simulink model "SURVEY_Simulations"  (R2021b)
settings: Solver=ode4  StartTime=0.0  StopTime=60  FixedStep=1e-3  RelTol=1e-3
(part 2 of 2)

== matlab function SURVEY_Simulations/Desired Trajectory ==
  data: t input; p_d output; dot_p_d output; ddot_p_d output; psi_d output; delta_p output; delta_eta output
function [p_d, dot_p_d, ddot_p_d, psi_d, delta_p, delta_eta] = fcn(t)
z0    = 0.3;
h     = 1.4;
%% Circunferencia
% ampx = 1;
% ampy = 1;
% ampz = 0.1;
% amps = 10*pi/180;
% frecx = 2*pi/5;
% frecy = 2*pi/5;
% frecz = 2*pi/5;
% frecs = 2*pi/5;

%% Lemniscata 1
% 
% ampx = 0.5;
% ampy = 1;
% ampz = 0.4;
% amps = 5*pi/180;
% frecx = 2*pi/4;
% frecy = 2*pi/8;
% frecz = 2*pi/4;
% frecs = 2*pi/4;
% 
% x_d      = ampx*sin(frecx*t);
% dot_x_d  = ampx*frecx*cos(frecx*t);
% ddot_x_d = -ampx*frecx^2*sin(frecx*t);
% 
% y_d      = ampy*cos(frecy*t);
% dot_y_d  = -ampy*frecy*sin(frecy*t);
% ddot_y_d = -ampy*frecy^2*cos(frecy*t);
% 
% if (t>=0 && t<=5)
%     z_d      = h - (h - z0)*exp(-ampz*t^3);
%     dot_z_d  = 3*ampz*t^2*(h - z0)*exp(-ampz*t^3);
%     ddot_z_d = (3*ampz*t^3 - 2)*3*ampz*t*(z0 - h)*exp(-ampz*t^3);
% else
%     z_d      = (h - ampz) + ampz*sin(frecz*t);
%     dot_z_d  = ampz*frecz*cos(frecz*t);
%     ddot_z_d = -ampz*frecz^2*sin(frecz*t);
% end
% 
% psi_d      = [amps*sin(frecs*t)
%               amps*frecs*cos(frecs*t)
%              -amps*frecs^2*sin(frecs*t)];
%        
% p_d      = [x_d; y_d; z_d];
% dot_p_d  = [dot_x_d; dot_y_d; dot_z_d];
% ddot_p_d = [ddot_x_d; ddot_y_d; ddot_z_d];

%% Lemniscata 2 (Experimento)

ampx = 0.5;
ampy = 1;
frecx = 2*pi/5;
frecy = frecx/2;
frecz = frecx;

x_d      = ampx*sin(frecx*t);
dot_x_d  = ampx*frecx*cos(frecx*t);
ddot_x_d = -ampx*frecx^2*sin(frecx*t);

y_d      = ampy*cos(frecy*t);
dot_y_d  = -ampy*frecy*sin(frecy*t);
ddot_y_d = -ampy*frecy^2*cos(frecy*t);

if (t>=0 && t<=5)
    z_d      = 1 - 0.7*exp(-0.1*t^3);
    dot_z_d  = 0.3*t^2*0.7*exp(-0.1*t^3);
    ddot_z_d = 0.3*0.7*(-0.1*3*exp(-0.1*t^3)*t^4 + 2*exp(-0.1*t^3)*t);
else
    z_d      = 1;
    dot_z_d  = 0;
    ddot_z_d = 0;
end

psi_d      = [0
              0
              0];
       
p_d      = [x_d; y_d; z_d];
dot_p_d  = [dot_x_d; dot_y_d; dot_z_d];
ddot_p_d = [ddot_x_d; ddot_y_d; ddot_z_d];

%% Disturbances
if (t>=40)
    delta_p = [0.5*sin(2*frecx*t)
               0.5*cos(2*frecy*t)
               0.5*sin(2*frecz*t)];

    d_eta = 0.045*sin(2.5*pi*t-3) + 0.09*sin(2*pi*t-7) + 0.135*sin(0.5*pi*t-9.5) + 0.09*sin(0.3*pi*t) + 0.054*sin(0.15*pi*t+4.5) + 0.045*sin(0.05*pi*t+2) + 0.135*sin(0.01*pi*t+3) + 0.225;
    delta_eta = [d_eta; d_eta; d_eta];
else
    delta_p = [0;0;0];
    delta_eta = [0;0;0];
end

== matlab function SURVEY_Simulations/Nonlinear PID-Type Controller/C. Posición ==
  data: ep input; Fz output; phi_d output; dot_ep input; int_ep input; ddot_p_d input; psi_d input; eta input; theta_d output
function [Fz,phi_d,theta_d] = fcn(ep,dot_ep,int_ep,ddot_p_d,psi_d,eta)
%--------------------------------------
m  = 1.82245;
g = 9.81;
%--------------------------------------
phi   = eta(1);
theta = eta(2);
gz    = [0;0;g];    
%--------------------------------------
Kpp = diag([9 9 11]);
Kdp = diag([6 6 6]);
Kip = diag([0.01 0.01 2.3]);
%-------------------------------------------------------------------
fp      = m*ddot_p_d + m*gz + Kpp*ep + Kip*int_ep +  Kdp*dot_ep;
theta_d = atan((fp(2)*sin(psi_d) + fp(1)*cos(psi_d))/fp(3));
phi_d   = atan(cos(theta_d)*(fp(1)*sin(psi_d) - fp(2)*cos(psi_d))/fp(3));
Fz      = fp(3)/(cos(phi)*cos(theta));
